simulink model "VIPLExit557TrgtPos"  (R2018b)
settings: Solver=FixedStepDiscrete  StartTime=0.0  StopTime=10.0  RelTol=1e-3
undefined symbols (not defined in the file or in its folder): arg, Rte_EEP_VIPLExitSecRwLtStBkReclnTrgtPos_Set, Rte_EEP_VIPLExitSecRwLtStCushFrntTrgtPos_Set, Rte_EEP_VIPLExitSecRwLtStFwdBkwdTrgtPos_Set, Rte_EEP_VIPLExitSecRwLtStLgrstInwdOtwdTrgtPos_Set, Rte_EEP_VIPLExitSecRwLtStLgrstUpwdDnwdTrgtPos_Set, Rte_EEP_VIPLExitThdRwLtStBkReclnTrgtPos_Set, Rte_EEP_VIPLExitThdRwLtStFwdBkwdTrgtPos_Set
settings Model: ModifiedHistory=2024.7.10 V3.0.0 557模式流程V1.9  Creator=sn2xws  LastModifiedBy=sn2xws
settings DataIOCC: SaveFormat=StructureWithTime
settings OptimizationCC: DefaultParameterBehavior=Inlined  EnhancedBackFolding=on  PassReuseOutputArgsAs=Individual arguments  ZeroExternalMemoryAtStartup=off  ZeroInternalMemoryAtStartup=off  OptimizeBlockOrder=speed  DifferentSizesBufferReuse=on  OptimizationCustomize=off
settings DebuggingCC: ParameterTunabilityLossMsg=error
settings SFSimCC: MATLABDynamicMemAlloc=off
settings RTWCC: SystemTargetFile=autosar.tlc  GenCodeOnly=on  TemplateMakefile=ert_default_tmf  Description=AUTOSAR  GenerateReport=on  IncludeHyperlinkInReport=on  LaunchReport=on  GenerateTraceInfo=on  GenerateTraceReport=on  GenerateTraceReportSl=on  GenerateTraceReportSf=on  GenerateTraceReportEml=on
settings CodeAppCC: ForceParamTrailComments=on  IgnoreCustomStorageClasses=off  OperatorAnnotations=on  SimulinkDataObjDesc=on  SFDataObjDesc=on  InsertBlockDesc=on
settings STFCustomTargetCC: TargetLangStandard=C99 (ISO)  MultiwordLength=256  ParMdlRefBuildCompliant=on  CompOptLevelCompliant=on  IncludeMdlTerminateFcn=off  CombineOutputUpdateFcns=on  SuppressErrorStatus=on  ERTCustomFileBanners=on  SupportNonFinite=off  SupportComplex=off  SupportContinuousTime=off  SupportNonInlinedSFcns=off  RemoveResetFunc=on  MATLABClassNameForMDSCustomization=Simulink.SoftwareTarget.ERTCustomization  AutosarCompliant=on  UseToolchainInfoCompliant=on  LookupTableObjectStructAxisOrder=2,1,3,4,...  LUTObjectStructOrderEvenSpacing=Size,Table,Breakpoints  SystemTargetFile=autosar.tlc
settings ERTTargetCC: TargetLangStandard=C99 (ISO)  ConcurrentExecutionCompliant=off  IncludeMdlTerminateFcn=off  SuppressErrorStatus=on  SupportNonFinite=off  SupportComplex=off  ModelStepFunctionPrototypeControlCompliant=off  CPPClassGenCompliant=off  AutosarCompliant=on  LookupTableObjectStructAxisOrder=2,1,3,4,...  LUTObjectStructOrderEvenSpacing=Size,Table,Breakpoints  InlinedParameterPlacement=NonHierarchical  ERTCustomFileTemplate=example_file_process.tlc  ERTFilePackagingFormat=Compact

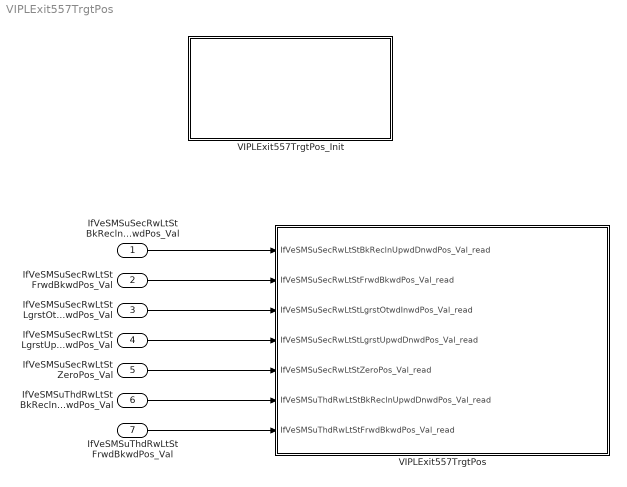
== system VIPLExit557TrgtPos ==
  IfVeSMSuSecRwLtStBkReclnUpwdDnwdPos_Val : Inport  OutDataTypeStr=uint16  PortDimensions=1
  IfVeSMSuSecRwLtStFrwdBkwdPos_Val : Inport  Port=2  OutDataTypeStr=uint16  PortDimensions=1
  IfVeSMSuSecRwLtStLgrstOtwdInwdPos_Val : Inport  Port=3  OutDataTypeStr=uint16  PortDimensions=1
  IfVeSMSuSecRwLtStLgrstUpwdDnwdPos_Val : Inport  Port=4  OutDataTypeStr=uint16  PortDimensions=1
  IfVeSMSuSecRwLtStZeroPos_Val : Inport  Port=5  OutDataTypeStr=uint16  PortDimensions=1
  IfVeSMSuThdRwLtStBkReclnUpwdDnwdPos_Val : Inport  Port=6  OutDataTypeStr=uint16  PortDimensions=1
  IfVeSMSuThdRwLtStFrwdBkwdPos_Val : Inport  Port=7  OutDataTypeStr=uint16  PortDimensions=1
  VIPLExit557TrgtPos : Subsystem
  VIPLExit557TrgtPos_Init : Subsystem
  wires:
  IfVeSMSuSecRwLtStBkReclnUpwdDnwdPos_Val/1 -> VIPLExit557TrgtPos/1(IfVeSMSuSecRwLtStBkReclnUpwdDnwdPos_Val_read)
  IfVeSMSuSecRwLtStFrwdBkwdPos_Val/1 -> VIPLExit557TrgtPos/2(IfVeSMSuSecRwLtStFrwdBkwdPos_Val_read)
  IfVeSMSuSecRwLtStLgrstOtwdInwdPos_Val/1 -> VIPLExit557TrgtPos/3(IfVeSMSuSecRwLtStLgrstOtwdInwdPos_Val_read)
  IfVeSMSuSecRwLtStLgrstUpwdDnwdPos_Val/1 -> VIPLExit557TrgtPos/4(IfVeSMSuSecRwLtStLgrstUpwdDnwdPos_Val_read)
  IfVeSMSuSecRwLtStZeroPos_Val/1 -> VIPLExit557TrgtPos/5(IfVeSMSuSecRwLtStZeroPos_Val_read)
  IfVeSMSuThdRwLtStBkReclnUpwdDnwdPos_Val/1 -> VIPLExit557TrgtPos/6(IfVeSMSuThdRwLtStBkReclnUpwdDnwdPos_Val_read)
  IfVeSMSuThdRwLtStFrwdBkwdPos_Val/1 -> VIPLExit557TrgtPos/7(IfVeSMSuThdRwLtStFrwdBkwdPos_Val_read)

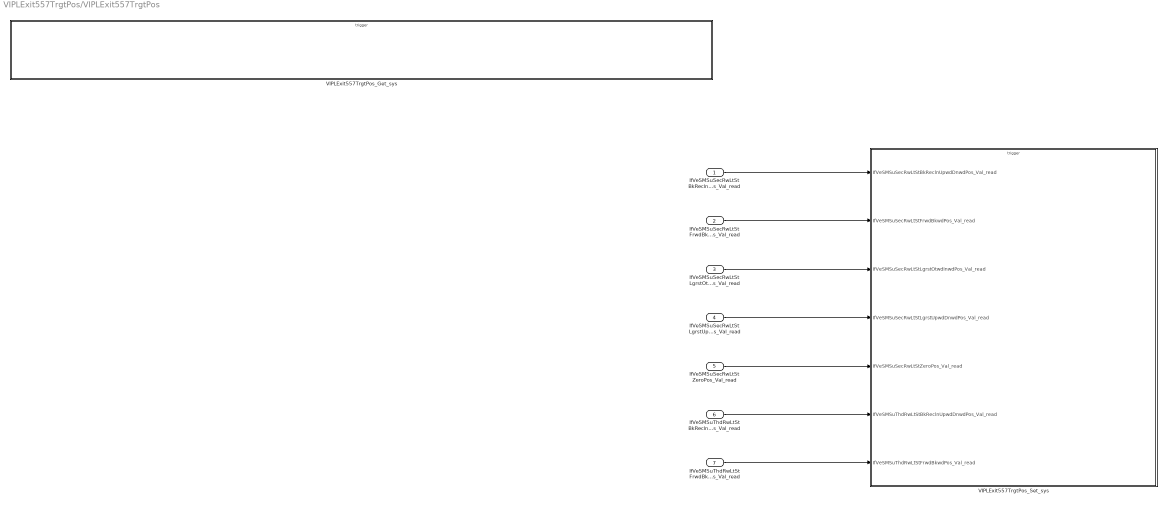
== system VIPLExit557TrgtPos/VIPLExit557TrgtPos ==
  IfVeSMSuSecRwLtStBkReclnUpwdDnwdPos_Val_read : Inport
  IfVeSMSuSecRwLtStFrwdBkwdPos_Val_read : Inport  Port=2
  IfVeSMSuSecRwLtStLgrstOtwdInwdPos_Val_read : Inport  Port=3
  IfVeSMSuSecRwLtStLgrstUpwdDnwdPos_Val_read : Inport  Port=4
  IfVeSMSuSecRwLtStZeroPos_Val_read : Inport  Port=5
  IfVeSMSuThdRwLtStBkReclnUpwdDnwdPos_Val_read : Inport  Port=6
  IfVeSMSuThdRwLtStFrwdBkwdPos_Val_read : Inport  Port=7
  VIPLExit557TrgtPos_Get_sys : Subsystem
  VIPLExit557TrgtPos_Set_sys : Subsystem
  wires:
  IfVeSMSuSecRwLtStBkReclnUpwdDnwdPos_Val_read/1 -> VIPLExit557TrgtPos_Set_sys/1(IfVeSMSuSecRwLtStBkReclnUpwdDnwdPos_Val_read)
  IfVeSMSuSecRwLtStFrwdBkwdPos_Val_read/1 -> VIPLExit557TrgtPos_Set_sys/2(IfVeSMSuSecRwLtStFrwdBkwdPos_Val_read)
  IfVeSMSuSecRwLtStLgrstOtwdInwdPos_Val_read/1 -> VIPLExit557TrgtPos_Set_sys/3(IfVeSMSuSecRwLtStLgrstOtwdInwdPos_Val_read)
  IfVeSMSuSecRwLtStLgrstUpwdDnwdPos_Val_read/1 -> VIPLExit557TrgtPos_Set_sys/4(IfVeSMSuSecRwLtStLgrstUpwdDnwdPos_Val_read)
  IfVeSMSuSecRwLtStZeroPos_Val_read/1 -> VIPLExit557TrgtPos_Set_sys/5(IfVeSMSuSecRwLtStZeroPos_Val_read)
  IfVeSMSuThdRwLtStFrwdBkwdPos_Val_read/1 -> VIPLExit557TrgtPos_Set_sys/7(IfVeSMSuThdRwLtStFrwdBkwdPos_Val_read)
  IfVeSMSuThdRwLtStBkReclnUpwdDnwdPos_Val_read/1 -> VIPLExit557TrgtPos_Set_sys/6(IfVeSMSuThdRwLtStBkReclnUpwdDnwdPos_Val_read)

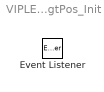
== system VIPLExit557TrgtPos/VIPLExit557TrgtPos_Init ==
  Event Listener : EventListener  EventName=reset

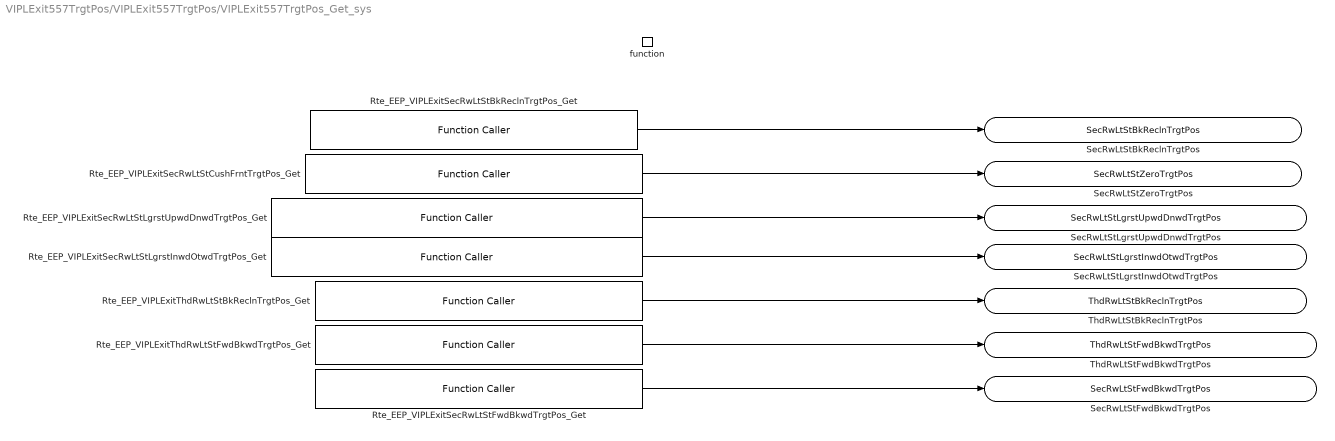
== system VIPLExit557TrgtPos/VIPLExit557TrgtPos/VIPLExit557TrgtPos_Get_sys ==
  function : TriggerPort  TriggerType=function-call  IsSimulinkFunction=on  FunctionName=VIPLExit557TrgtPos_Get  VariantControl=(inherit)
  Rte_EEP_VIPLExitSecRwLtStBkReclnTrgtPos_Get : FunctionCaller  FunctionPrototype=arg = Rte_EEP_VIPLExitSecRwLtStBkReclnTrgtPos_Get()  OutputArgumentSpecifications=P_EEP_Uint16
  Rte_EEP_VIPLExitSecRwLtStCushFrntTrgtPos_Get : FunctionCaller  FunctionPrototype=arg = Rte_EEP_VIPLExitSecRwLtStCushFrntTrgtPos_Get()  OutputArgumentSpecifications=P_EEP_Uint16
  Rte_EEP_VIPLExitSecRwLtStFwdBkwdTrgtPos_Get : FunctionCaller  FunctionPrototype=arg = Rte_EEP_VIPLExitSecRwLtStFwdBkwdTrgtPos_Get()  OutputArgumentSpecifications=P_EEP_Uint16
  Rte_EEP_VIPLExitSecRwLtStLgrstInwdOtwdTrgtPos_Get : FunctionCaller  FunctionPrototype=arg = Rte_EEP_VIPLExitSecRwLtStLgrstInwdOtwdTrgtPos_Get()  OutputArgumentSpecifications=P_EEP_Uint16
  Rte_EEP_VIPLExitSecRwLtStLgrstUpwdDnwdTrgtPos_Get : FunctionCaller  FunctionPrototype=arg = Rte_EEP_VIPLExitSecRwLtStLgrstUpwdDnwdTrgtPos_Get()  OutputArgumentSpecifications=P_EEP_Uint16
  Rte_EEP_VIPLExitThdRwLtStBkReclnTrgtPos_Get : FunctionCaller  FunctionPrototype=arg = Rte_EEP_VIPLExitThdRwLtStBkReclnTrgtPos_Get()  OutputArgumentSpecifications=P_EEP_Uint16
  Rte_EEP_VIPLExitThdRwLtStFwdBkwdTrgtPos_Get : FunctionCaller  FunctionPrototype=arg = Rte_EEP_VIPLExitThdRwLtStFwdBkwdTrgtPos_Get()  OutputArgumentSpecifications=P_EEP_Uint16
  SecRwLtStBkReclnTrgtPos : ArgOut  OutDataTypeStr=uint16  ArgumentName=SecRwLtStBkReclnTrgtPos
  SecRwLtStZeroTrgtPos : ArgOut  Port=2  OutDataTypeStr=uint16  ArgumentName=SecRwLtStZeroTrgtPos
  SecRwLtStLgrstUpwdDnwdTrgtPos : ArgOut  Port=3  OutDataTypeStr=uint16  ArgumentName=SecRwLtStLgrstUpwdDnwdTrgtPos
  SecRwLtStLgrstInwdOtwdTrgtPos : ArgOut  Port=4  OutDataTypeStr=uint16  ArgumentName=SecRwLtStLgrstInwdOtwdTrgtPos
  ThdRwLtStBkReclnTrgtPos : ArgOut  Port=5  OutDataTypeStr=uint16  ArgumentName=ThdRwLtStBkReclnTrgtPos
  ThdRwLtStFwdBkwdTrgtPos : ArgOut  Port=6  OutDataTypeStr=uint16  ArgumentName=ThdRwLtStFwdBkwdTrgtPos
  SecRwLtStFwdBkwdTrgtPos : ArgOut  Port=7  OutDataTypeStr=uint16  ArgumentName=SecRwLtStFwdBkwdTrgtPos
  wires:
  Rte_EEP_VIPLExitSecRwLtStBkReclnTrgtPos_Get/1 -> SecRwLtStBkReclnTrgtPos/1
  Rte_EEP_VIPLExitSecRwLtStCushFrntTrgtPos_Get/1 -> SecRwLtStZeroTrgtPos/1
  Rte_EEP_VIPLExitSecRwLtStLgrstUpwdDnwdTrgtPos_Get/1 -> SecRwLtStLgrstUpwdDnwdTrgtPos/1
  Rte_EEP_VIPLExitSecRwLtStLgrstInwdOtwdTrgtPos_Get/1 -> SecRwLtStLgrstInwdOtwdTrgtPos/1
  Rte_EEP_VIPLExitThdRwLtStBkReclnTrgtPos_Get/1 -> ThdRwLtStBkReclnTrgtPos/1
  Rte_EEP_VIPLExitThdRwLtStFwdBkwdTrgtPos_Get/1 -> ThdRwLtStFwdBkwdTrgtPos/1
  Rte_EEP_VIPLExitSecRwLtStFwdBkwdTrgtPos_Get/1 -> SecRwLtStFwdBkwdTrgtPos/1

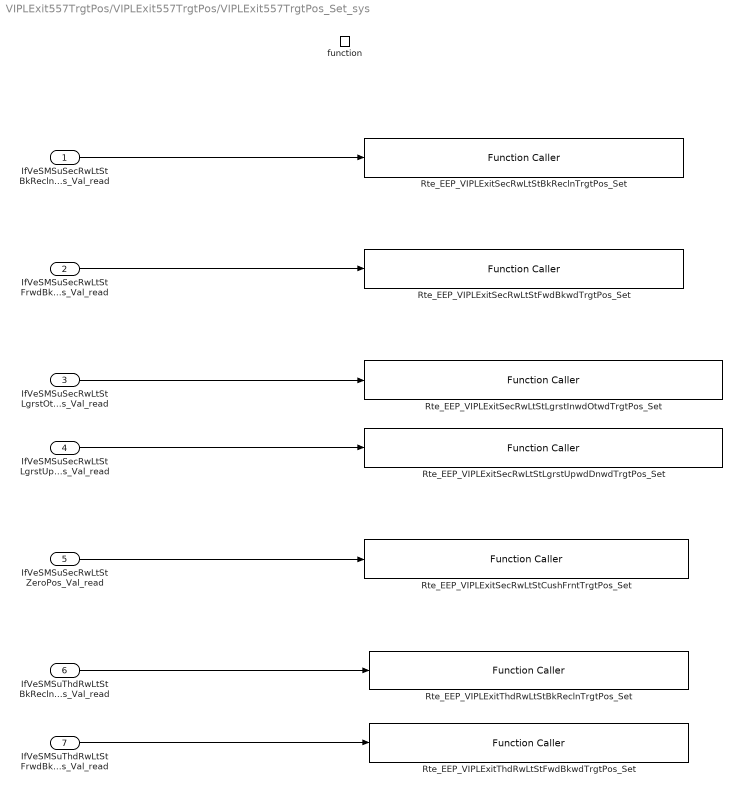
== system VIPLExit557TrgtPos/VIPLExit557TrgtPos/VIPLExit557TrgtPos_Set_sys ==
  IfVeSMSuSecRwLtStBkReclnUpwdDnwdPos_Val_read : Inport
  IfVeSMSuSecRwLtStFrwdBkwdPos_Val_read : Inport  Port=2
  IfVeSMSuSecRwLtStLgrstOtwdInwdPos_Val_read : Inport  Port=3
  IfVeSMSuSecRwLtStLgrstUpwdDnwdPos_Val_read : Inport  Port=4
  IfVeSMSuSecRwLtStZeroPos_Val_read : Inport  Port=5
  IfVeSMSuThdRwLtStBkReclnUpwdDnwdPos_Val_read : Inport  Port=6
  IfVeSMSuThdRwLtStFrwdBkwdPos_Val_read : Inport  Port=7
  function : TriggerPort  TriggerType=function-call  IsSimulinkFunction=on  FunctionName=VIPLExit557TrgtPos_Set  VariantControl=(inherit)
  Rte_EEP_VIPLExitSecRwLtStBkReclnTrgtPos_Set : FunctionCaller  FunctionPrototype=Rte_EEP_VIPLExitSecRwLtStBkReclnTrgtPos_Set(arg)  InputArgumentSpecifications=P_EEP_Uint16
  Rte_EEP_VIPLExitSecRwLtStCushFrntTrgtPos_Set : FunctionCaller  FunctionPrototype=Rte_EEP_VIPLExitSecRwLtStCushFrntTrgtPos_Set(arg)  InputArgumentSpecifications=P_EEP_Uint16
  Rte_EEP_VIPLExitSecRwLtStFwdBkwdTrgtPos_Set : FunctionCaller  FunctionPrototype=Rte_EEP_VIPLExitSecRwLtStFwdBkwdTrgtPos_Set(arg)  InputArgumentSpecifications=P_EEP_Uint16
  Rte_EEP_VIPLExitSecRwLtStLgrstInwdOtwdTrgtPos_Set : FunctionCaller  FunctionPrototype=Rte_EEP_VIPLExitSecRwLtStLgrstInwdOtwdTrgtPos_Set(arg)  InputArgumentSpecifications=P_EEP_Uint16
  Rte_EEP_VIPLExitSecRwLtStLgrstUpwdDnwdTrgtPos_Set : FunctionCaller  FunctionPrototype=Rte_EEP_VIPLExitSecRwLtStLgrstUpwdDnwdTrgtPos_Set(arg)  InputArgumentSpecifications=P_EEP_Uint16
  Rte_EEP_VIPLExitThdRwLtStBkReclnTrgtPos_Set : FunctionCaller  FunctionPrototype=Rte_EEP_VIPLExitThdRwLtStBkReclnTrgtPos_Set(arg)  InputArgumentSpecifications=P_EEP_Uint16
  Rte_EEP_VIPLExitThdRwLtStFwdBkwdTrgtPos_Set : FunctionCaller  FunctionPrototype=Rte_EEP_VIPLExitThdRwLtStFwdBkwdTrgtPos_Set(arg)  InputArgumentSpecifications=P_EEP_Uint16
  wires:
  IfVeSMSuSecRwLtStBkReclnUpwdDnwdPos_Val_read/1 -> Rte_EEP_VIPLExitSecRwLtStBkReclnTrgtPos_Set/1
  IfVeSMSuSecRwLtStFrwdBkwdPos_Val_read/1 -> Rte_EEP_VIPLExitSecRwLtStFwdBkwdTrgtPos_Set/1
  IfVeSMSuSecRwLtStLgrstOtwdInwdPos_Val_read/1 -> Rte_EEP_VIPLExitSecRwLtStLgrstInwdOtwdTrgtPos_Set/1
  IfVeSMSuSecRwLtStLgrstUpwdDnwdPos_Val_read/1 -> Rte_EEP_VIPLExitSecRwLtStLgrstUpwdDnwdTrgtPos_Set/1
  IfVeSMSuSecRwLtStZeroPos_Val_read/1 -> Rte_EEP_VIPLExitSecRwLtStCushFrntTrgtPos_Set/1
  IfVeSMSuThdRwLtStBkReclnUpwdDnwdPos_Val_read/1 -> Rte_EEP_VIPLExitThdRwLtStBkReclnTrgtPos_Set/1
  IfVeSMSuThdRwLtStFrwdBkwdPos_Val_read/1 -> Rte_EEP_VIPLExitThdRwLtStFwdBkwdTrgtPos_Set/1
